simulink model "PartC"  (R2019b)
settings: Solver=VariableStepAuto  StartTime=0.0  StopTime=10.0  RelTol=1e-3
PreLoadFcn:
  | load AllBuses
settings Model: Creator=Lenovo  LastModifiedBy=Lenovo
settings OptimizationCC: DefaultParameterBehavior=Inlined

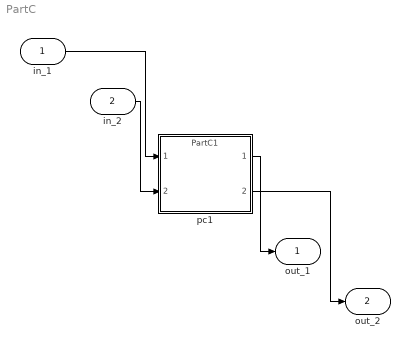
== system PartC ==
  in_1 : Inport  OutDataTypeStr=double
  in_2 : Inport  Port=2  OutDataTypeStr=int32
  pc1 : ModelReference  ModelNameDialog=PartC1  SimulationMode=Normal  ModelReferenceVersion=1.1
  out_1 : Outport  OutDataTypeStr=double
  out_2 : Outport  Port=2  OutDataTypeStr=boolean
  wires:
  in_1/1 -> pc1/1
  in_2/1 -> pc1/2
  pc1/1 -> out_1/1
  pc1/2 -> out_2/1
